simulink model "PID_Controller_v1"  (R2019a)
settings: Solver=VariableStepAuto  StartTime=0.0  StopTime=inf  RelTol=1e-3
libraries: instrumentlib x2, simulink x1
settings Model: Creator=facuolmed_o  LastModifiedBy=facuolmed_o

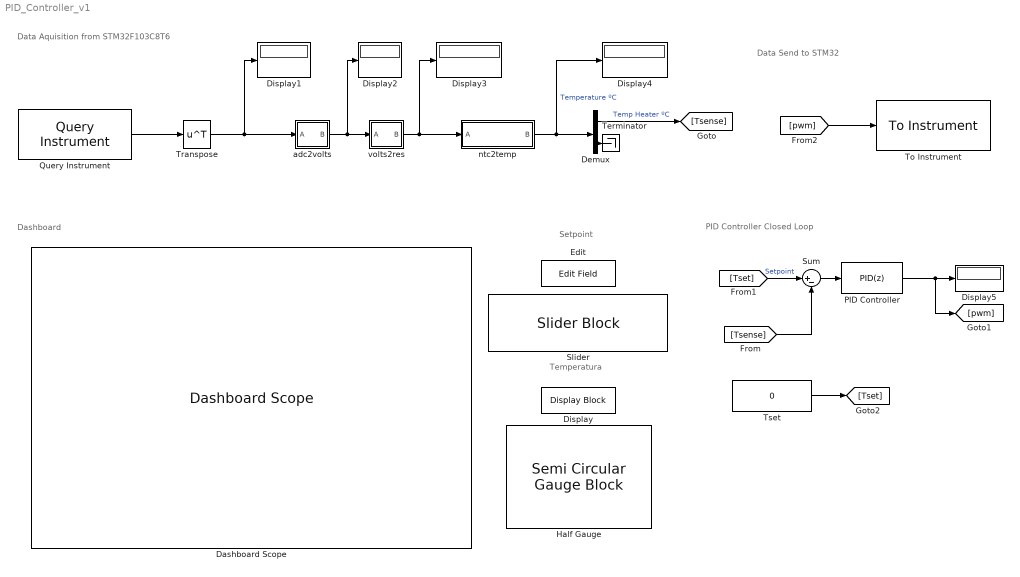
== system PID_Controller_v1 ==
  note: Data Send to STM32
  note: Dashboard
  note: PID Controller Closed Loop
  note: Temperatura
  note: Setpoint
  note: Data Aquisition from STM32F103C8T6
  Dashboard Scope : DashboardScope  TimeSpan=1000  Ymax=400  ScaleAtStop=off
  Demux : Demux  Outputs=2
  Display : DisplayBlock  LabelPosition=Hide  Format=short
  Display{1..5} (5 alike) : Display
      Display1 settings: Format=bank
      Display2 settings: Format=bank
      Display3 settings: Format=bank
      Display4 settings: Format=bank
  Edit : EditField  LabelPosition=Hide  ShowInitialText=on  Alignment=Center
  Half Gauge : SemiCircularGaugeBlock  ScaleMax=400
  PID Controller : simulink/Continuous/PID Controller  Controller=PID  Form=Parallel  TimeDomain=Discrete-time  SampleTime=0.8  IntegratorMethod=Forward Euler  FilterMethod=Forward Euler  ControllerParametersSource=internal  P=10  I=0.003  D=0.7  UseFilter=off  N=100  TunerSelectOption=Transfer Function Based (PID Tuner App)  InitialConditionSource=internal  InitialConditionForIntegrator=0  InitialConditionForFilter=0  DifferentiatorICPrevScaledInput=0  ExternalReset=none  TrackingMode=off  Kt=1  LimitOutput=on  UpperSaturationLimit=255  LowerSaturationLimit=0  LinearizeAsGain=on  AntiWindupMode=none  Kb=1  POutMin=[]  POutMax=[]  IOutMin=[]  IOutMax=[]  DOutMin=[]  DOutMax=[]  NOutMin=[]  NOutMax=[]  SumOutMin=[]  SumOutMax=[]  SaturationOutMin=[]  SaturationOutMax=[]  PParamMin=[]  PParamMax=[]  IParamMin=[]  IParamMax=[]  DParamMin=[]  DParamMax=[]  NParamMin=[]  NParamMax=[]  KbParamMin=[]  KbParamMax=[]  KtParamMin=[]  KtParamMax=[]  KbOutMin=[]  KbOutMax=[]  KtOutMin=[]  KtOutMax=[]  IntegratorOutMin=[]  IntegratorOutMax=[]  FilterOutMin=[]  FilterOutMax=[]  SumI1OutMin=[]  SumI1OutMax=[]  SumI2OutMin=[]  SumI2OutMax=[]  SumI3OutMin=[]  SumI3OutMax=[]  SumI4OutMin=[]  SumI4OutMax=[]  SumDOutMin=[]  SumDOutMax=[]  DifferentiatorOutMin=[]  DifferentiatorOutMax=[]  FilterDiffOutCoefMin=[]  FilterDiffOutCoefMax=[]  ReciprocalOutMin=[]  ReciprocalOutMax=[]  SumDenOutMin=[]  SumDenOutMax=[]  SumNumOutMin=[]  SumNumOutMax=[]  DivideOutMin=[]  DivideOutMax=[]  IntegratorContinuousStateAttributes=''  IntegratorStateMustResolveToSignalObject=off  IntegratorRTWStateStorageClass=Auto  FilterContinuousStateAttributes=''  FilterStateMustResolveToSignalObject=off  FilterRTWStateStorageClass=Auto  ParallelPVariant=InternalParameters  IdealPVariant=Disabled  IVariant=InternalParameters  DVariant=InternalParameters  IntegratorVariant=Discrete  SatVariant=Enabled  AWVariant=Passthrough  PCopyVariant=Disabled  TRVariant=Disabled  FdbkBlocksVariant=Forward  IdealPFdbkVariant=Disabled  SatFdbkVariant=Disabled  DerivativeFilterVariant=Differentiator  NVariant=Passthrough  NCopyVariant=Disabled_SignalSpec  FilterICVariant=InternalICsDifferentiator  IntegratorICVariant=InternalICs  ExternalResetVariant=Disabled  TRSumVariant=Passthrough  SumFdbkVariant=Disabled  SumVariant=Sum_PID
  Query Instrument : instrumentlib/Query Instrument  sampleTime=0  isWorkspaceObject=off  timeout=10  inputBufferSize=512  protocol=Serial  serialPort=COM2  baudRate=115200  gpibVendor=Keysight Technologies  boardIndex=0  primaryAddress=1  secondaryAddress=0  visaVendor=Keysight  visaSerialPort=0  chassisIndex=0  logicalAddress=0  tcpRemoteHost='127.0.0.1'  tcpRemotePort=4500  udpRemoteHost='127.0.0.1'  udpRemotePort=9090  visaTCPBoardIndex=0  visaTCPRemoteHost='127.0.0.1'  usbBoardIndex=0  usbManufID=0  usbModelCode=0  usbSerialNumber=0  initAction=None  initCommand='DATA:SOURCE CH1'  initFunction=get  queryCommand=''  responseFormat=ASCII  asciiFormatting='%d,%d\n'  precision=8-bit unsigned integer  byteOrder=Little endian  valuesToRead=1  removeBytes=off  afterOutputAction=Repeat query for new data  enableFrames=on  frameSize=2
      settings: SourceProductName=Instrument Control Toolbox  SourceProductBaseCode=IC
  Slider : SliderBlock  ScaleMax=255
  Sum : Sum  Inputs=|+-
  Terminator : Terminator
  To Instrument : instrumentlib/To Instrument  sampleTime=0  isWorkspaceObject=off  timeout=10  inputBufferSize=100  protocol=Serial  serialPort=COM2  baudRate=115200  gpibVendor=ICS Electronics  boardIndex=0  primaryAddress=1  secondaryAddress=0  visaVendor=Keysight  visaSerialPort=0  chassisIndex=0  logicalAddress=0  tcpRemoteHost='127.0.0.1'  tcpRemotePort=4500  udpRemoteHost='127.0.0.1'  udpRemotePort=9090  visaTCPBoardIndex=0  visaTCPRemoteHost='127.0.0.1'  usbBoardIndex=0  usbManufID=0  usbModelCode=0  usbSerialNumber=0  initAction=None  initCommand='DATA:SOURCE CH1'  initFunction=get  command=''  sendFormat=Binary  asciiFormatting='%c'  precision=8-bit unsigned integer  byteOrder=Little endian
      settings: SourceProductName=Instrument Control Toolbox  SourceProductBaseCode=IC
  Transpose : Math  Operator=transpose  SaturateOnIntegerOverflow=on
  "Tset " : Constant  Value=0  OutDataTypeStr=double  SampleTime=0
  adc2volts : Subsystem
  ntc2temp : Subsystem
  volts2res : Subsystem
  wires:
  Query Instrument/1 -> Transpose/1
  Transpose/1 -> Display1/1, adc2volts/1(A)
  "Tset "/1 -> [Tset]
  adc2volts/1(B) -> volts2res/1(A), Display2/1
  volts2res/1(B) -> ntc2temp/1(A), Display3/1
  Demux/1 -> [Tsense]  "Temp Heater ºC"
  Sum/1 -> PID Controller/1
  [Tset] -> Sum/1  "Setpoint"
  [Tsense] -> Sum/2
  ntc2temp/1(B) -> Display4/1, Demux/1  "Temperature ºC"
  PID Controller/1 -> Display5/1, [pwm]
  [pwm] -> To Instrument/1
  Demux/2 -> Terminator/1

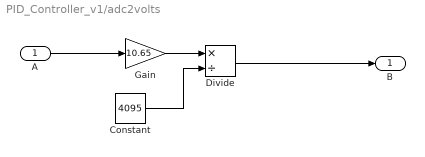
== system PID_Controller_v1/adc2volts ==
  A : Inport
  Constant : Constant  Value=4095
  Divide : Product  Inputs=*/
  Gain : Gain  Gain=10.65
  B : Outport
  wires:
  A/1 -> Gain/1
  Gain/1 -> Divide/1
  Divide/1 -> B/1
  Constant/1 -> Divide/2

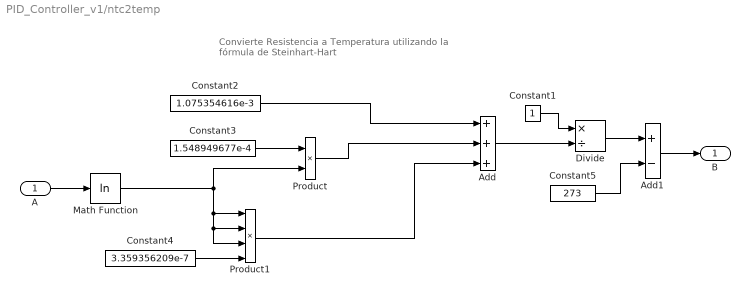
== system PID_Controller_v1/ntc2temp ==
  note: Convierte Resistencia a Temperatura utilizando la fórmula de Steinhart-Hart
  A : Inport
  Add : Sum  Inputs=+++
  Add1 : Sum  Inputs=+-
  Constant1 : Constant
  Constant2 : Constant  Value=1.075354616e-3
  Constant3 : Constant  Value=1.548949677e-4
  Constant4 : Constant  Value=3.359356209e-7
  Constant5 : Constant  Value=273
  Divide : Product  Inputs=*/
  Math Function : Math  Operator=log  SaturateOnIntegerOverflow=on
  Product : Product
  Product1 : Product  Inputs=4
  B : Outport
  wires:
  Constant1/1 -> Divide/1
  A/1 -> Math Function/1
  Constant2/1 -> Add/1
  Constant3/1 -> Product/1
  Math Function/1 -> Product1/3, Product1/2, Product1/1, Product/2
  Product/1 -> Add/2
  Add/1 -> Divide/2
  Constant4/1 -> Product1/4
  Product1/1 -> Add/3
  Divide/1 -> Add1/1
  Constant5/1 -> Add1/2
  Add1/1 -> B/1

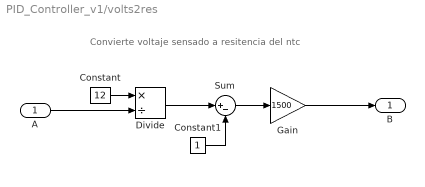
== system PID_Controller_v1/volts2res ==
  note: Convierte voltaje sensado a resitencia del ntc
  A : Inport
  Constant : Constant  Value=12
  Constant1 : Constant
  Divide : Product  Inputs=*/
  Gain : Gain  Gain=1500
  Sum : Sum  Inputs=|+-
  B : Outport
  wires:
  Constant/1 -> Divide/1
  A/1 -> Divide/2
  Divide/1 -> Sum/1
  Constant1/1 -> Sum/2
  Sum/1 -> Gain/1
  Gain/1 -> B/1
